simulink model "Controller_cruise"  (R2020a)
settings: Solver=VariableStepAuto  StartTime=0.0  StopTime=10.0  RelTol=1e-3
values from neighbouring files (symbols this model uses):
  b = 50.0    [cruise_datadict.sldd]
  m = 1000.0    [cruise_datadict.sldd]
settings Model: DataDictionary=cruise_datadict.sldd  Creator=kiran  LastModifiedBy=kiran
settings DataIOCC: SaveOutput=off  SaveTime=off

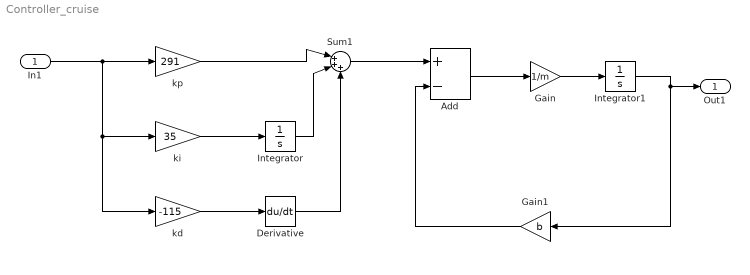
== system Controller_cruise ==
  In1 : Inport  OutDataTypeStr=double  PortDimensions=1  SampleTime=0
  Add : Sum  Inputs=+-
  Derivative : Derivative
  Gain : Gain  Gain=1/m
  Gain1 : Gain  Gain=b
  Integrator : Integrator
  Integrator1 : Integrator
  Sum1 : Sum  Inputs=|+++
  kd : Gain  Gain=-115
  ki : Gain  Gain=35
  kp : Gain  Gain=291
  Out1 : Outport  OutDataTypeStr=double  PortDimensions=1  SampleTime=0
  wires:
  In1/1 -> ki/1, kd/1, kp/1
  Add/1 -> Gain/1
  Gain1/1 -> Add/2
  Derivative/1 -> Sum1/3
  kp/1 -> Sum1/1
  Integrator/1 -> Sum1/2
  ki/1 -> Integrator/1
  Sum1/1 -> Add/1
  kd/1 -> Derivative/1
  Gain/1 -> Integrator1/1
  Integrator1/1 -> Gain1/1, Out1/1
